simulink model "SiDrivetrain"  (R2017b)
settings: Solver=ode23tb  StartTime=0.0  StopTime=50  RelTol=1e-3  EnableMultiTasking=on
model workspace (MAT data in the model file):
  N = [-4.7 4.75 4.75 3.75 3.25 2.75 2.25 1.5 1 0.75]
  Ndiff = 3
  Re = 0.3
  b_axle = Simulink.Parameter
  b_axle.Value = 10
  b_axle.DataType = 'auto'
  b_axle.Dimensions = [1 1]
  b_driveshaft = Simulink.Parameter
  b_driveshaft.Value = 10
  b_driveshaft.DataType = 'auto'
  b_driveshaft.Dimensions = [1 1]
  dt_DCT = Simulink.Parameter
  dt_DCT.Value = 0.001
  dt_DCT.DataType = 'auto'
  dt_DCT.Dimensions = [1 1]
  k_axle = Simulink.Parameter
  k_axle.Value = 5000
  k_axle.DataType = 'auto'
  k_axle.Dimensions = [1 1]
  k_driveshaft = Simulink.Parameter
  k_driveshaft.Value = 1000
  k_driveshaft.DataType = 'auto'
  k_driveshaft.Dimensions = [1 1]
  k_hyd = Simulink.Parameter
  k_hyd.Value = 5000000
  k_hyd.DataType = 'auto'
  k_hyd.Dimensions = [1 1]
  tau_hyd = Simulink.Parameter
  tau_hyd.Value = 0.01
  tau_hyd.DataType = 'auto'
  tau_hyd.Dimensions = [1 1]
  wc_shaft = Simulink.Parameter
  wc_shaft.Value = 300
  wc_shaft.DataType = 'auto'
  wc_shaft.Dimensions = [1 1]
values from neighbouring files (symbols this model uses):
  b_axle = 10.0    [DrivetrainEvDD.sldd]    (also in DrivetrainHevMmDD.sldd; SiDrivetrainDD.sldd)
  b_driveshaft = 10.0    [DrivetrainEvDD.sldd]    (also in DrivetrainHevMmDD.sldd; SiDrivetrainDD.sldd)
  k_axle = 5000.0    [DrivetrainEvDD.sldd]    (also in DrivetrainHevMmDD.sldd; SiDrivetrainDD.sldd)
  k_driveshaft = 1000.0    [DrivetrainEvDD.sldd]    (also in DrivetrainHevMmDD.sldd; SiDrivetrainDD.sldd)
libraries: autolibsharedcoupling x12, autolibshared x7, autolibshareddiff x4, autolibutils x3, autolibcoupling x2, simulink x2, autolibsharedtransfixedgear x2, autolibtransdct x1, autolibshareddrivetraincommon x1, autolibtranscontrols x1
(part 1 of 5)
settings Model: ModifiedByFormat=The MathWorks, Inc.  PauseTimes=9  Creator=The MathWorks, Inc.  LastModifiedBy=The MathWorks, Inc.
settings DataIOCC: DSMLogging=off
settings DebuggingCC: UnderspecifiedInitializationDetection=Classic  MergeDetectMultiDrivingBlocksExec=none
settings ModelReferenceCC: PropagateSignalLabelsOutOfModel=off
settings CodeAppCC: StateflowObjectComments=on
settings GRTTargetCC: TargetLangStandard=C89/C90 (ANSI)
settings ConfigComp: CovMetricSettings=dsw  CovHtmlReporting=on  CovSaveCumulativeToWorkspaceVar=on  CovSaveSingleToWorkspaceVar=on  CovShowResultsExplorer=off  CovExternalEMLEnable=off
settings SimscapeCC: SimscapeNormalizeSystem=off  SimscapeNominalValues={1, 'bar'; 1, 'cm^3/s'; 1, 'bar*kg/s'; 1, 'kJ/kg'; 1, 'kW'; }

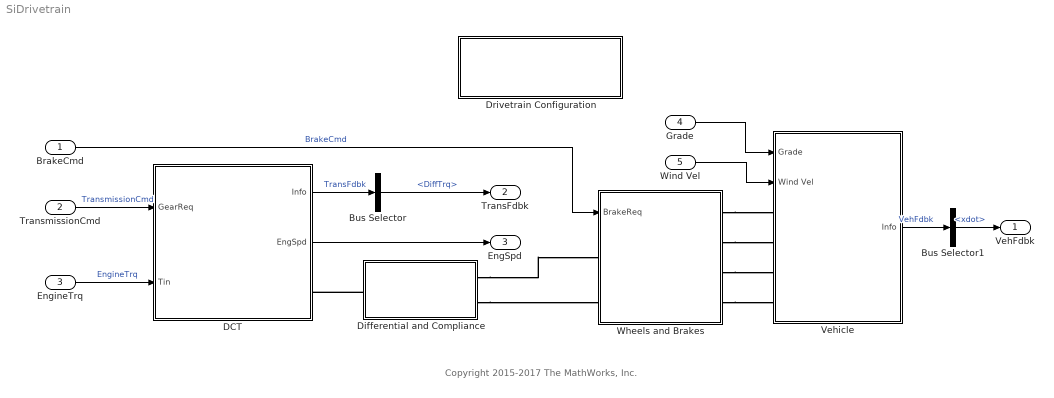
== system SiDrivetrain ==
  note: Copyright 2015-2017 The MathWorks, Inc.
  BrakeCmd : Inport
  TransmissionCmd : Inport  Port=2
  EngineTrq : Inport  Port=3
  Grade : Inport  Port=4
  Wind Vel : Inport  Port=5
  Bus Selector : BusSelector  OutputSignals=Diff.DiffTrq
  Bus Selector1 : BusSelector  OutputSignals=BdyFrm.Cg.Vel.xdot
  DCT : Subsystem  Variant=on  OverrideUsingVariant=0
  Differential and Compliance : Subsystem  Variant=on  OverrideUsingVariant=0
  Drivetrain Configuration : Subsystem  mask(Drivetrain Configuration){drivetrainMode=Front Wheel Drive}
      mask prompts: drivetrainMode "Drivetrain Mode"
      mask help: Use this block to configure the dirvetrain mode.
      settings: AttributesFormatString=Active Mode: %<drivetrainMode>
      mask TypeOptions drivetrainMode: Front Wheel Drive | Rear Wheel Drive | All Wheel Drive
      mask Callback drivetrainMode:
      | switch get_param(gcb,'drivetrainMode')
      |     case 'Front Wheel Drive'
      |         set_param([bdroot '/Wheels and Brakes'],'OverrideUsingVariant','0')
      |         set_param([bdroot '/Differential and Compliance'],'OverrideUsingVariant','0')
      |     case 'Rear Wheel Drive'
      |         set_param([bdroot '/Wheels and Brakes'],'OverrideUsingVariant','1')
      |         set_param([bdroot '/Differential and Compliance'],'OverrideUsingVariant','1')
      |     case 'All Wheel Drive'
      |         set_param([bdroot '/Wheels and Brakes'],'OverrideUsingVariant','2')
      |         set_param([bdroot '/Differential and Compliance'],'OverrideUsingVariant','2')
      |     otherwise
      |         set_param([bdroot '/Wheels and Brakes'],'OverrideUsingVariant','0')
      |         set_param([bdroot '/Differential and Compliance'],'OverrideUsingVariant','0')
      | end
      mask Display: disp('Double click to configure drivetrain')
  Vehicle : Subsystem
  Wheels and Brakes : Subsystem  Variant=on  OverrideUsingVariant=0
  VehFdbk : Outport
  TransFdbk : Outport  Port=2  BusOutputAsStruct=on
  EngSpd : Outport  Port=3  BusOutputAsStruct=on
  wires:
  Vehicle/1(Info) -> Bus Selector1/1  "VehFdbk"
  BrakeCmd/1 -> Wheels and Brakes/1(BrakeReq)  "BrakeCmd"
  Bus Selector1/1 -> VehFdbk/1  "<xdot>"
  Bus Selector/1 -> TransFdbk/1  "<DiffTrq>"
  TransmissionCmd/1 -> DCT/1(GearReq)  "TransmissionCmd"
  DCT/1(Info) -> Bus Selector/1  "TransFdbk"
  DCT/2(EngSpd) -> EngSpd/1
  EngineTrq/1 -> DCT/2(Tin)  "EngineTrq"
  Grade/1 -> Vehicle/1(Grade)
  Wind Vel/1 -> Vehicle/2(Wind Vel)
  connections:
  Wheels and Brakes/RConn1 -- Vehicle/LConn1
  Differential and Compliance/RConn1 -- Wheels and Brakes/LConn1
  Differential and Compliance/LConn1 -- DCT/RConn1
  Wheels and Brakes/RConn2 -- Vehicle/LConn2
  Wheels and Brakes/RConn3 -- Vehicle/LConn3
  Wheels and Brakes/RConn4 -- Vehicle/LConn4
  Differential and Compliance/RConn2 -- Wheels and Brakes/LConn2

== system SiDrivetrain/DCT ==
  note: 1) Add Subsystem or Model blocks as valid variant choices.
      | 2) You cannot connect blocks at this level. At simulation, connectivity is automatically
      | determined, based on the active variant and port name matching.
  GearReq : Inport
  Tin : Inport  Port=2
  DCT Block : Subsystem  VariantControl=0
      settings: MinAlgLoopOccurrences=on
  DCT System : Subsystem  VariantControl=1
      settings: MinAlgLoopOccurrences=on
  T : PMIOPort  Port=1  Side=Right
  Info : Outport
  EngSpd : Outport  Port=2

== system SiDrivetrain/Differential and Compliance ==
  All Wheel Drive : Subsystem  VariantControl=2
  Front Wheel Drive : Subsystem  VariantControl=0
  Rear Wheel Drive : Subsystem  VariantControl=1
  D : PMIOPort  Port=1  Side=Left
  A1 : PMIOPort  Port=2  Side=Right
  A2 : PMIOPort  Port=3  Side=Right

== system SiDrivetrain/Drivetrain Configuration ==

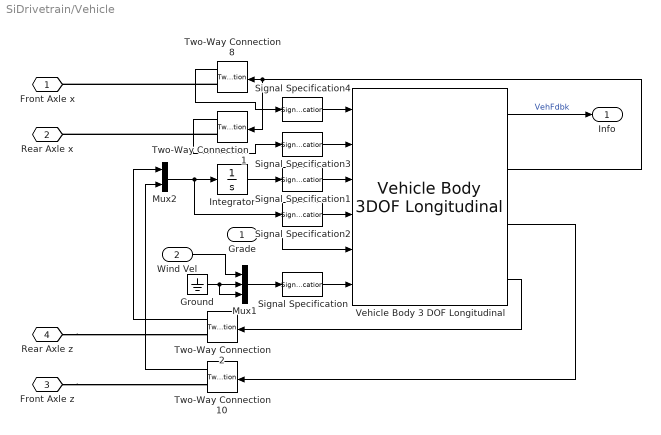
== system SiDrivetrain/Vehicle ==
  Grade : Inport  Unit=deg
  Wind Vel : Inport  Port=2  Unit=m/s
  Ground : Ground
  Integrator : Integrator
  Mux1 : Mux  Inputs=3
  Mux2 : Mux  Inputs=2
  Signal Specification : SignalSpecification  Unit=m/s
  Signal Specification1 : SignalSpecification  Unit=m
  Signal Specification2 : SignalSpecification  Unit=m/s
  Signal Specification3 : SignalSpecification  Unit=N
  Signal Specification4 : SignalSpecification  Unit=N
  Two-Way Connection{1..2,8,10} (4 alike) : TwoWayConnection
  Vehicle Body 3 DOF Longitudinal : autolibshared/Vehicle Body 3DOF Longitudinal  VariantControl=SL  groundType=Axle displacement, velocity  NF=2  NR=2  m=1200  a=1.4  b=1.8  h=.35  Cd=.3  Af=2  x_o=0  xdot_o=0  Cl=.1  z_o=-.35  zdot_o=0  Iyy=3000  Cpm=.1  theta_o=0  q_o=0  FskF=[-50, -1, 0, 2, 3, 52].*1.25e4  dzsF=[-5e-3, -1e-4, 0, .2, .2001, .2051]  FsbF=[-10000 -100 -10 0 10 100 10000]  dzdotsF=[-10 -1 -.1 0 .1 1 10]  FskR=[-50, -1, 0, 2, 3, 52].*7.5e3  dzsR=[-5e-3, -1e-4, 0, .2, .2001, .2051]  FsbR=[-10000 -100 -10 0 10 100 10000]  dzdotsR=[-10 -1 -.1 0 .1 1 10]  Pabs=101325  T=273  g=9.81  blkID=0
      settings: SourceProductName=Powertrain Blockset  SourceProductBaseCode=PW
  Front Axle x : PMIOPort  Port=1  Side=Left
  Rear Axle x : PMIOPort  Port=2  Side=Left
  Front Axle z : PMIOPort  Port=3  Side=Left
  Rear Axle z : PMIOPort  Port=4  Side=Left
  Info : Outport
  wires:
  Vehicle Body 3 DOF Longitudinal/3 -> Two-Way Connection10/1
  Vehicle Body 3 DOF Longitudinal/2 -> Two-Way Connection1/1, Two-Way Connection8/1
  Two-Way Connection8/1 -> Signal Specification4/1
  Vehicle Body 3 DOF Longitudinal/1 -> Info/1  "VehFdbk"
  Ground/1 -> Mux1/2, Mux1/3
  Mux1/1 -> Signal Specification/1
  Two-Way Connection1/1 -> Signal Specification3/1
  Vehicle Body 3 DOF Longitudinal/4 -> Two-Way Connection2/1
  Two-Way Connection2/1 -> Mux2/1
  Two-Way Connection10/1 -> Mux2/2
  Mux2/1 -> Integrator/1, Signal Specification2/1
  Integrator/1 -> Signal Specification1/1
  Wind Vel/1 -> Mux1/1
  Grade/1 -> Vehicle Body 3 DOF Longitudinal/5
  Signal Specification/1 -> Vehicle Body 3 DOF Longitudinal/6
  Signal Specification1/1 -> Vehicle Body 3 DOF Longitudinal/3
  Signal Specification2/1 -> Vehicle Body 3 DOF Longitudinal/4
  Signal Specification3/1 -> Vehicle Body 3 DOF Longitudinal/2
  Signal Specification4/1 -> Vehicle Body 3 DOF Longitudinal/1
  connections:
  Two-Way Connection8/RConn1 -- Front Axle x/RConn1
  Front Axle z/RConn1 -- Two-Way Connection10/RConn1
  Two-Way Connection1/RConn1 -- Rear Axle x/RConn1
  Rear Axle z/RConn1 -- Two-Way Connection2/RConn1

== system SiDrivetrain/Wheels and Brakes ==
  BrakeReq : Inport
  All Wheel Drive : Subsystem  VariantControl=2
  Front Wheel Drive : Subsystem  VariantControl=0
  Rear Wheel Drive : Subsystem  VariantControl=1
  Front Axle x : PMIOPort  Port=1  Side=Right
  Axle Torque 1 : PMIOPort  Port=2  Side=Left
  Rear Axle x : PMIOPort  Port=3  Side=Right
  Front Axle z : PMIOPort  Port=4  Side=Right
  Rear Axle z : PMIOPort  Port=5  Side=Right
  Axle Torque 2 : PMIOPort  Port=6  Side=Left

== system SiDrivetrain/DCT/DCT Block ==
  GearReq : Inport
  Tin : Inport  Port=2
  Driveshaft Compliance : autolibsharedcoupling/Torsional Compliance  port_config=Two-way connection  k=k_driveshaft  b=b_driveshaft  theta_o=0  domega_o=0  omega_c=wc_shaft  blkID=0
      settings: SourceProductName=Powertrain Blockset
  Dual Clutch Transmission : autolibtransdct/Dual Clutch Transmission  VariantControl=0  cntrlType=Ideal integrated controller  Jin=0.2  bin=.001  omegain_o=0  G=[-1, 0, 1, 2, 3, 4, 5, 6, 7, 8]  N=N  Jout=[0.28 0.28 0.28 0.24 0.2 0.18 0.11 0.11 0.11 0.11]  bout=[.001 .001 .001 .0025 .002 .001 .001 .001 .001 .001]  eta=[0.930, 0.930, 0.930, 0.940,0.947, 0.948,0.946, 0.943,0.940, 0.935 ]  omegaout_o=0  G_o=0  tauc=.01  ts=.02  tc=.5  R=.25  K_c=2.5e3  mus=0.3  muk=0.25  ClutchLocked=off  SynchLocked=off  maxAbsSpd=5e3
      settings: SourceProductName=Powertrain Blockset  SourceProductBaseCode=PW
  Two-Way Connection2 : TwoWayConnection
  T : PMIOPort  Port=1  Side=Right
  Info : Outport
  EngSpd : Outport  Port=2
  wires:
  Dual Clutch Transmission/1 -> Info/1
  Dual Clutch Transmission/2 -> EngSpd/1
  GearReq/1 -> Dual Clutch Transmission/1
  Dual Clutch Transmission/3 -> Two-Way Connection2/1
  Tin/1 -> Dual Clutch Transmission/2
  Two-Way Connection2/1 -> Dual Clutch Transmission/3
  connections:
  T/RConn1 -- Driveshaft Compliance/RConn1
  Driveshaft Compliance/LConn1 -- Two-Way Connection2/RConn1

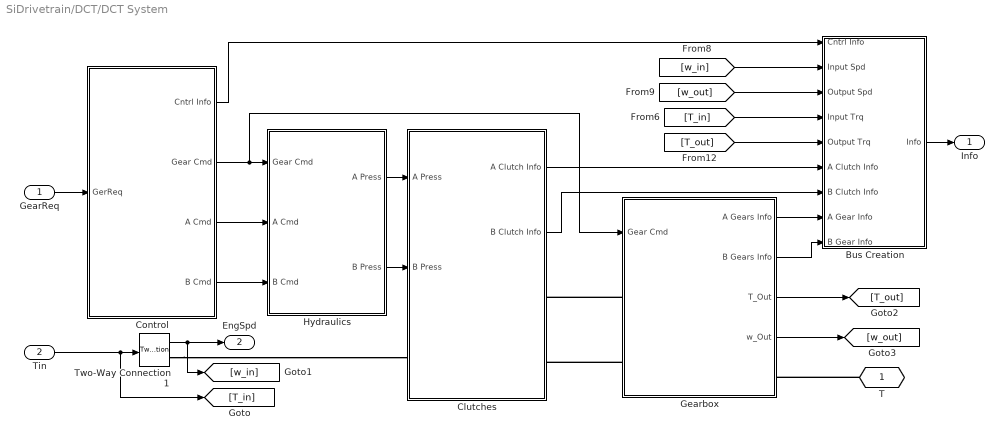
== system SiDrivetrain/DCT/DCT System ==
  GearReq : Inport
  Tin : Inport  Port=2  Unit=N*m
  Bus Creation : Subsystem
  Clutches : Subsystem
  Control : Subsystem
  Gearbox : Subsystem
  Hydraulics : Subsystem
  Two-Way Connection1 : TwoWayConnection
  T : PMIOPort  Port=1  Side=Right
  Info : Outport
  EngSpd : Outport  Port=2  Unit=rad/s
  wires:
  Tin/1 -> [T_in], Two-Way Connection1/1
  Two-Way Connection1/1 -> [w_in], EngSpd/1
  Gearbox/1(A Gears Info) -> Bus Creation/8(A Gear Info)
  Gearbox/2(B Gears Info) -> Bus Creation/9(B Gear Info)
  Clutches/1(A Clutch Info) -> Bus Creation/6(A Clutch Info)
  Clutches/2(B Clutch Info) -> Bus Creation/7(B Clutch Info)
  Hydraulics/1(A Press) -> Clutches/1(A Press)
  Hydraulics/2(B Press) -> Clutches/2(B Press)
  Control/2(Gear Cmd) -> Hydraulics/1(Gear Cmd), Gearbox/1(Gear Cmd)
  GearReq/1 -> Control/1(GerReq)
  Control/3(A Cmd) -> Hydraulics/2(A Cmd)
  Control/4(B Cmd) -> Hydraulics/3(B Cmd)
  [T_out] -> Bus Creation/5(Output Trq)
  [T_in] -> Bus Creation/4(Input Trq)
  Control/1(Cntrl Info) -> Bus Creation/1(Cntrl Info)
  [w_out] -> Bus Creation/3(Output Spd)
  [w_in] -> Bus Creation/2(Input Spd)
  Bus Creation/1(Info) -> Info/1
  Gearbox/3(T_Out) -> [T_out]
  Gearbox/4(w_Out) -> [w_out]
  connections:
  T/RConn1 -- Gearbox/RConn1
  Gearbox/LConn1 -- Clutches/RConn1
  Two-Way Connection1/RConn1 -- Clutches/LConn1
  Gearbox/LConn2 -- Clutches/RConn2

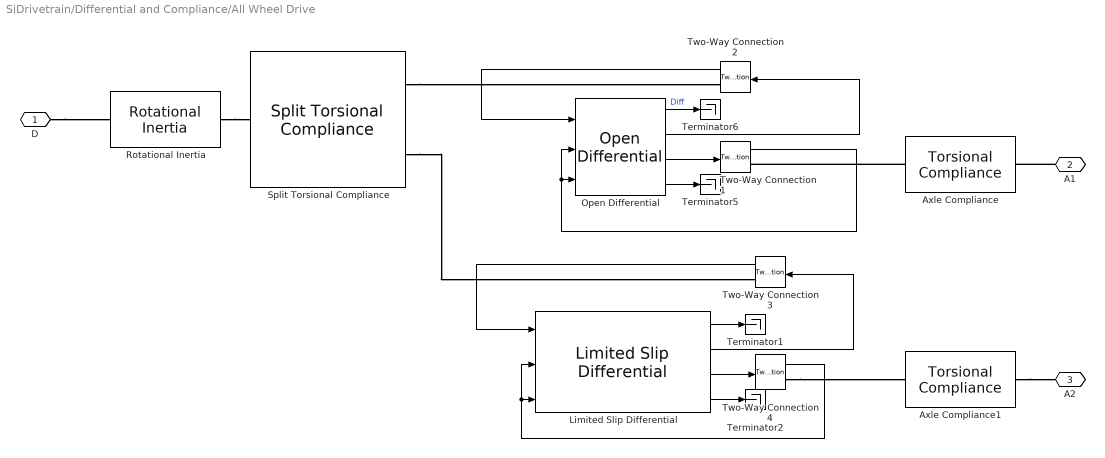
== system SiDrivetrain/Differential and Compliance/All Wheel Drive ==
  Axle Compliance : autolibsharedcoupling/Torsional Compliance  port_config=Two-way connection  k=k_axle  b=b_axle  theta_o=0  domega_o=0  omega_c=wc_shaft  blkID=0
      settings: SourceProductName=Powertrain Blockset
  Axle Compliance1 : autolibsharedcoupling/Torsional Compliance  port_config=Two-way connection  k=k_axle  b=b_axle  theta_o=0  domega_o=0  omega_c=wc_shaft  blkID=0
      settings: SourceProductName=Powertrain Blockset
  Limited Slip Differential : autolibshareddiff/Limited Slip Differential  shaftSwitchMask=To the left of center-line  Ndiff=Ndiff  Jd=.025  bd=1e-3  Jw1=.01  bw1=1e-3  Jw2=.01  bw2=1e-3  omegaw1o=0  omegaw2o=0  couplingType=Pre-loaded ideal clutch  Ndisks=4  Reff=.20  Fc=500  muc=[.16 0.13 0.115 0.11 0.105 0.1025 0.10125]  dw=[0 10 20 40 60 80 100]  IdealInterpMethod=Linear  IdealExtrapMethod=Linear  Tdw=[-100, -90, -50, -5, 0, 5, 50, 90, 100]  dwT=[-200, -175, -100, - 50, 0, 50, 100, 175, 200]  TdwInterpMethod=Linear  TdwExtrapMethod=Linear  TTin=[-200 -175 -100 - 50 0 50 100 175 200]  Tin=[-200 -175 -100 - 50 0 50 100 175 200]  TTinInterpMethod=Linear  TTinExtrapMethod=Linear  tauC=.01  maxAbsSpd=5e3
      settings: SourceProductName=Powertrain Blockset  SourceProductBaseCode=PW
  Open Differential : autolibshareddiff/Open Differential  shaftSwitchMask=To the left of center-line  Ndiff=Ndiff  Jd=.025  bd=1e-3  Jw1=.01  bw1=1e-3  Jw2=.01  bw2=1e-3  omegaw1o=0  omegaw2o=0  maxAbsSpd=5e3
      settings: SourceProductName=Powertrain Blockset
  Rotational Inertia : autolibsharedcoupling/Rotational Inertia  port_config=Two-way connection  J=.01  b=.001  omega_o=0  externJ=off  blkID=0
      settings: SourceProductName=Powertrain Blockset  SourceProductBaseCode=PW
  Split Torsional Compliance : autolibsharedcoupling/Split Torsional Compliance  port_config=Two-way connection  cplrMode=Shaft split  k1=5e4  b1=1e2  omega1_c=3000  theta1_o=0  domega1_o=0  k2=5e4  b2=1e2  omega2_c=3000  theta2_o=0  domega2_o=0  blkID=0
      settings: SourceProductName=Powertrain Blockset  SourceProductBaseCode=PW
  Terminator{1..2,5..6} (4 alike) : Terminator
  Two-Way Connection{1..4} (4 alike) : TwoWayConnection
  D : PMIOPort  Port=1  Side=Left
  A1 : PMIOPort  Port=2  Side=Right
  A2 : PMIOPort  Port=3  Side=Right
  wires:
  Open Differential/1 -> Terminator6/1  "Diff"
  Two-Way Connection2/1 -> Open Differential/1
  Two-Way Connection1/1 -> Open Differential/2, Open Differential/3
  Open Differential/3 -> Two-Way Connection1/1
  Open Differential/4 -> Terminator5/1
  Open Differential/2 -> Two-Way Connection2/1
  Two-Way Connection3/1 -> Limited Slip Differential/1
  Limited Slip Differential/1 -> Terminator1/1
  Limited Slip Differential/3 -> Two-Way Connection4/1
  Two-Way Connection4/1 -> Limited Slip Differential/3, Limited Slip Differential/2
  Limited Slip Differential/2 -> Two-Way Connection3/1
  Limited Slip Differential/4 -> Terminator2/1
  connections:
  D/RConn1 -- Rotational Inertia/LConn1
  Split Torsional Compliance/RConn1 -- Two-Way Connection2/RConn1
  Axle Compliance/LConn1 -- Two-Way Connection1/RConn1
  A1/RConn1 -- Axle Compliance/RConn1
  Split Torsional Compliance/RConn2 -- Two-Way Connection3/RConn1
  Axle Compliance1/RConn1 -- A2/RConn1
  Two-Way Connection4/RConn1 -- Axle Compliance1/LConn1
  Rotational Inertia/RConn1 -- Split Torsional Compliance/LConn1

== system SiDrivetrain/Differential and Compliance/Front Wheel Drive ==
  Axle Compliance : autolibsharedcoupling/Torsional Compliance  port_config=Two-way connection  k=k_axle  b=b_axle  theta_o=0  domega_o=0  omega_c=wc_shaft  blkID=0
      settings: SourceProductName=Powertrain Blockset
  Open Differential : autolibshareddiff/Open Differential  shaftSwitchMask=To the left of center-line  Ndiff=Ndiff  Jd=.025  bd=1e-3  Jw1=.01  bw1=1e-3  Jw2=.01  bw2=1e-3  omegaw1o=0  omegaw2o=0  maxAbsSpd=5e3
      settings: SourceProductName=Powertrain Blockset
  Terminator5 : Terminator
  Terminator6 : Terminator
  Two-Way Connection1 : TwoWayConnection
  Two-Way Connection2 : TwoWayConnection
  D : PMIOPort  Port=1  Side=Left
  A1 : PMIOPort  Port=2  Side=Right
  wires:
  Open Differential/1 -> Terminator6/1  "Diff"
  Two-Way Connection2/1 -> Open Differential/1
  Two-Way Connection1/1 -> Open Differential/2, Open Differential/3
  Open Differential/3 -> Two-Way Connection1/1
  Open Differential/4 -> Terminator5/1
  Open Differential/2 -> Two-Way Connection2/1
  connections:
  A1/RConn1 -- Axle Compliance/RConn1
  Axle Compliance/LConn1 -- Two-Way Connection1/RConn1
  Two-Way Connection2/RConn1 -- D/RConn1

== system SiDrivetrain/Differential and Compliance/Rear Wheel Drive ==
  Axle Compliance : autolibsharedcoupling/Torsional Compliance  port_config=Two-way connection  k=k_axle  b=b_axle  theta_o=0  domega_o=0  omega_c=wc_shaft  blkID=0
      settings: SourceProductName=Powertrain Blockset
  Open Differential : autolibshareddiff/Open Differential  shaftSwitchMask=To the left of center-line  Ndiff=Ndiff  Jd=.025  bd=1e-3  Jw1=.01  bw1=1e-3  Jw2=.01  bw2=1e-3  omegaw1o=0  omegaw2o=0  maxAbsSpd=5e3
      settings: SourceProductName=Powertrain Blockset
  Terminator5 : Terminator
  Terminator6 : Terminator
  Two-Way Connection1 : TwoWayConnection
  Two-Way Connection2 : TwoWayConnection
  D : PMIOPort  Port=1  Side=Left
  A1 : PMIOPort  Port=2  Side=Right
  wires:
  Open Differential/1 -> Terminator6/1  "Diff"
  Two-Way Connection2/1 -> Open Differential/1
  Two-Way Connection1/1 -> Open Differential/2, Open Differential/3
  Open Differential/3 -> Two-Way Connection1/1
  Open Differential/4 -> Terminator5/1
  Open Differential/2 -> Two-Way Connection2/1
  connections:
  A1/RConn1 -- Axle Compliance/RConn1
  Axle Compliance/LConn1 -- Two-Way Connection1/RConn1
  Two-Way Connection2/RConn1 -- D/RConn1
